simulink model "ADC_tb_sd"  (Simulink 7.3)
settings: Solver=ode45  StartTime=4  StopTime=7.95  RelTol=1e-3
libraries: simulink x1
settings Model: Creator=jamshaid  LastModifiedBy=jamsjaid
settings DataIOCC: MaxDataPoints=2000
settings OptimizationCC: InitFltsAndDblsToZero=on
settings DebuggingCC: SaveWithParameterizedLinksMsg=none
settings GRTTargetCC: TargetFcnLib=ansi_tfl_tmw.mat

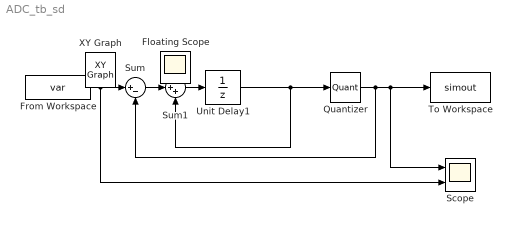
== system ADC_tb_sd ==
  From Workspace : FromWorkspace  VariableName=var  SampleTime=0.004
  Quantizer : Quantizer  QuantizationInterval=1
  Scope : Scope  NumInputPorts=2
      settings: YMin=-5~-5  YMax=5~5
  Sum : Sum  Inputs=|+-  OutDataType=sfix(16)  OutScaling=2^0
  Sum1 : Sum  Inputs=|++  OutDataType=sfix(16)  OutScaling=2^0
  To Workspace : ToWorkspace  VariableName=simout  SampleTime=-1  SaveFormat=Array
  Unit Delay1 : UnitDelay  SampleTime=-1
  Floating Scope : Scope
      settings: Floating=on
  XY Graph : simulink/Sinks/XY Graph  IOType=viewer  SystemSampleTime=-1  xmin=-1  xmax=1  ymin=-1  ymax=1  st=-1
  wires:
  Sum1/1 -> Unit Delay1/1
  Sum/1 -> Sum1/1
  Unit Delay1/1 -> Sum1/2, Quantizer/1
  Quantizer/1 -> Sum/2, To Workspace/1, Scope/1
  From Workspace/1 -> Sum/1, Scope/2
